simulink model "simu"  (R2021a)
settings: Solver=VariableStepAuto  StartTime=0.0  StopTime=10  RelTol=1e-3
values from neighbouring files (symbols this model uses):
  A = -25.77    [desarrollo.m]
  B = 2876    [desarrollo.m]
  C = 1    [desarrollo.m]
  K = 1.32    [desarrollo.m]
  Kd = acker(Aad,Bad,z)    [desarrollo.m]
  Ts = 0.05    [desarrollo.m]
undefined symbols (not defined in the file or in its folder): den, DiscIntNeverNeededParam, num
settings Model: Creator=pierr  LastModifiedBy=pierr

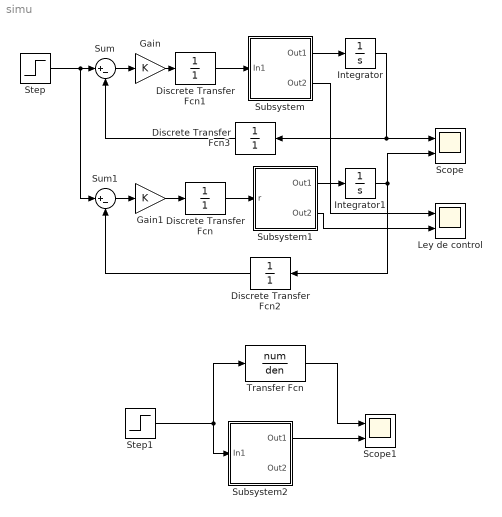
== system simu ==
  Discrete Transfer Fcn{,1..3} (4 alike) : DiscreteTransferFcn  Denominator=[1]
  Gain : Gain  Gain=K
  Gain1 : Gain  Gain=K
  Integrator : Integrator
  Integrator1 : Integrator
  Ley de control : Scope  NumInputPorts=2
  Scope : Scope  NumInputPorts=2
  Scope1 : Scope  NumInputPorts=2
  Step : Step  Time=0  After=100  SampleTime=Ts
  Step1 : Step  Time=0  After=100  SampleTime=Ts
  Subsystem : Subsystem
  Subsystem1 : Subsystem
  Subsystem2 : Subsystem
  Sum : Sum  Inputs=|+-
  Sum1 : Sum  Inputs=|+-
  Transfer Fcn : TransferFcn  Numerator=num  Denominator=den
  wires:
  Sum/1 -> Gain/1
  Subsystem/1(Out1) -> Integrator/1
  Step/1 -> Sum1/1, Sum/1
  Sum1/1 -> Gain1/1
  Subsystem1/1(Out1) -> Integrator1/1
  Integrator/1 -> Discrete Transfer Fcn3/1, Scope/1
  Integrator1/1 -> Discrete Transfer Fcn2/1, Scope/2
  Step1/1 -> Transfer Fcn/1, Subsystem2/1(In1)
  Transfer Fcn/1 -> Scope1/1
  Gain/1 -> Discrete Transfer Fcn1/1
  Discrete Transfer Fcn1/1 -> Subsystem/1(In1)
  Gain1/1 -> Discrete Transfer Fcn/1
  Discrete Transfer Fcn/1 -> Subsystem1/1(r)
  Discrete Transfer Fcn2/1 -> Sum1/2
  Discrete Transfer Fcn3/1 -> Sum/2
  Subsystem/2(Out2) -> Ley de control/1
  Subsystem1/2(Out2) -> Ley de control/2
  Subsystem2/1(Out1) -> Scope1/2

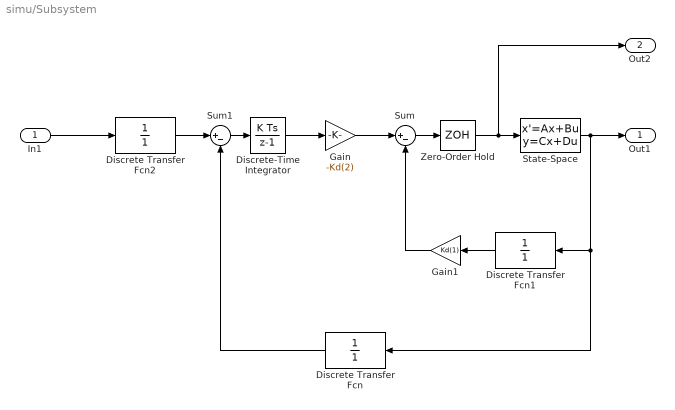
== system simu/Subsystem ==
  In1 : Inport
  Discrete Transfer Fcn : DiscreteTransferFcn  Denominator=[1]  SampleTime=Ts
  Discrete Transfer Fcn1 : DiscreteTransferFcn  Denominator=[1]  SampleTime=Ts
  Discrete Transfer Fcn2 : DiscreteTransferFcn  Denominator=[1]  SampleTime=Ts
  Discrete-Time Integrator : DiscreteIntegrator  SampleTime=Ts  ICPrevOutput=DiscIntNeverNeededParam  ICPrevScaledInput=DiscIntNeverNeededParam
  Gain : Gain  Gain=-Kd(2)
  Gain1 : Gain  Gain=Kd(1)
  State-Space : StateSpace  A=A  B=B  C=C  D=0  InitialCondition=0
  Sum : Sum  Inputs=|+-
  Sum1 : Sum  Inputs=|+-
  Zero-Order Hold : ZeroOrderHold  SampleTime=Ts
  Out1 : Outport
  Out2 : Outport  Port=2
  wires:
  Discrete Transfer Fcn/1 -> Sum1/2
  Sum1/1 -> Discrete-Time Integrator/1
  State-Space/1 -> Out1/1, Discrete Transfer Fcn/1, Discrete Transfer Fcn1/1
  Discrete-Time Integrator/1 -> Gain/1
  Discrete Transfer Fcn1/1 -> Gain1/1
  Gain/1 -> Sum/1
  Gain1/1 -> Sum/2
  Sum/1 -> Zero-Order Hold/1
  Zero-Order Hold/1 -> Out2/1, State-Space/1
  In1/1 -> Discrete Transfer Fcn2/1
  Discrete Transfer Fcn2/1 -> Sum1/1

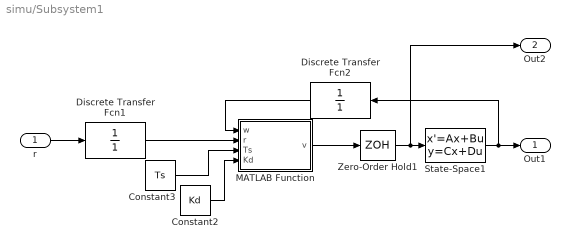
== system simu/Subsystem1 ==
  r : Inport
  Constant2 : Constant  Value=Kd
  Constant3 : Constant  Value=Ts
  Discrete Transfer Fcn1 : DiscreteTransferFcn  Denominator=[1]  SampleTime=Ts
  Discrete Transfer Fcn2 : DiscreteTransferFcn  Denominator=[1]  SampleTime=Ts
  MATLAB Function : MATLAB Function  TreatAsAtomicUnit=on
  State-Space1 : StateSpace  A=A  B=B  C=C  D=0  InitialCondition=0
  Zero-Order Hold1 : ZeroOrderHold  SampleTime=Ts
  Out1 : Outport
  Out2 : Outport  Port=2
  wires:
  MATLAB Function/1(v) -> Zero-Order Hold1/1
  Zero-Order Hold1/1 -> Out2/1, State-Space1/1
  Constant3/1 -> MATLAB Function/3(Ts)
  State-Space1/1 -> Out1/1, Discrete Transfer Fcn2/1
  Discrete Transfer Fcn2/1 -> MATLAB Function/1(w)
  Constant2/1 -> MATLAB Function/4(Kd)
  r/1 -> Discrete Transfer Fcn1/1
  Discrete Transfer Fcn1/1 -> MATLAB Function/2(r)

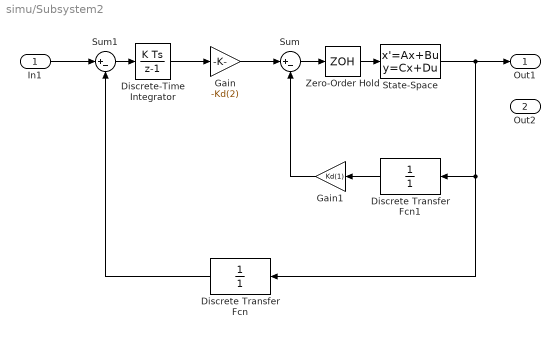
== system simu/Subsystem2 ==
  In1 : Inport
  Discrete Transfer Fcn : DiscreteTransferFcn  Denominator=[1]  SampleTime=Ts
  Discrete Transfer Fcn1 : DiscreteTransferFcn  Denominator=[1]  SampleTime=Ts
  Discrete-Time Integrator : DiscreteIntegrator  SampleTime=Ts  ICPrevOutput=DiscIntNeverNeededParam  ICPrevScaledInput=DiscIntNeverNeededParam
  Gain : Gain  Gain=-Kd(2)
  Gain1 : Gain  Gain=Kd(1)
  State-Space : StateSpace  A=A  B=B  C=C  D=0  InitialCondition=0
  Sum : Sum  Inputs=|+-
  Sum1 : Sum  Inputs=|+-
  Zero-Order Hold : ZeroOrderHold  SampleTime=Ts
  Out1 : Outport
  Out2 : Outport  Port=2
  wires:
  Discrete Transfer Fcn/1 -> Sum1/2
  Sum1/1 -> Discrete-Time Integrator/1
  State-Space/1 -> Out1/1, Discrete Transfer Fcn/1, Discrete Transfer Fcn1/1
  Discrete-Time Integrator/1 -> Gain/1
  Discrete Transfer Fcn1/1 -> Gain1/1
  Gain/1 -> Sum/1
  Gain1/1 -> Sum/2
  Sum/1 -> Zero-Order Hold/1
  Zero-Order Hold/1 -> State-Space/1
  In1/1 -> Sum1/1

== matlab function simu/Subsystem1/MATLAB Function ==
  settings: updateMethod=DISCRETE
  data: w input; v output; r input; Ts input; Kd input
function v = fcn(w,r,Ts,Kd)

persistent ek_1
persistent x2_1
if isempty (ek_1)
    ek_1=0;
    x2_1=0;
end
ek=r-w;
x2=x2_1+Ts/2*(ek+ek_1);
v = -Kd(1)*w-Kd(2)*x2;

ek_1=ek;
x2_1=x2;
